simulink library "Mech_Hydro_Elec_Multibody_Lib"  (R2021b)
settings: Solver=ode45  StartTime=0.0  StopTime=10.0  RelTol=1e-3  EnableMultiTasking=on
libraries: fl_ps_legacy_lib x27, fl_lib x24, mech_hydro_forcesPS_lib x21, sm_lib x15, $bdroot x4
(part 2 of 2)

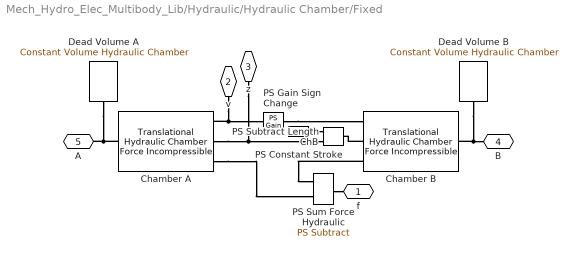
== system Mech_Hydro_Elec_Multibody_Lib/Hydraulic/Hydraulic Chamber/Fixed ==
  Chamber A : mech_hydro_forcesPS_lib/Hydraulic/Translational Hydraulic Chamber Force Incompressible  area=area_A m^2  q_specify=off  q_priority=None  q=0 m^3/s  q_nominal_specify=off  q_nominal_unit=m^3/s  q_nominal_value=1
      settings: InternalSimscapePortConfiguration="{\"Bottom\":[],\"Left\":[{\"id\":\"velocity\",\"label\":\"v\",\"type\":\"input\"},{\"id\":\"position\",\"label\":\"p\",\"type\":\"input\"},{\"id\":\"force\",\"label\":\"f\",\"type\":\"output\"}],\"Right\":[{\"id\":\"A\",\"label\":\"A\",\"type\":\"foundation.hydraulic.hydraulic\"}],\"Top\":[]}"
  Chamber B : mech_hydro_forcesPS_lib/Hydraulic/Translational Hydraulic Chamber Force Incompressible  area=area_B m^2  q_specify=off  q_priority=None  q=0 m^3/s  q_nominal_specify=off  q_nominal_unit=m^3/s  q_nominal_value=1
      settings: InternalSimscapePortConfiguration="{\"Bottom\":[],\"Left\":[{\"id\":\"velocity\",\"label\":\"v\",\"type\":\"input\"},{\"id\":\"position\",\"label\":\"p\",\"type\":\"input\"},{\"id\":\"force\",\"label\":\"f\",\"type\":\"output\"}],\"Right\":[{\"id\":\"A\",\"label\":\"A\",\"type\":\"foundation.hydraulic.hydraulic\"}],\"Top\":[]}"
  Dead Volume A : fl_lib/Hydraulic/Hydraulic Elements/Constant Volume Hydraulic Chamber  ch_sp=1  wall_type=1  ch_volume=dead_vol_A m^3  d_in=1e-2 m  length=1 m  pr_r_coef=1.2e-12 m/Pa  time_const=0.01 s  k_sh=1.4  pressure_specify=off  pressure_priority=High  pressure=0 Pa  pressure_nominal_specify=off  pressure_nominal_unit=Pa  pressure_nominal_value=1  diameter_incr_specify=off  diameter_incr_priority=High  diameter_incr=0 m  diameter_incr_nominal_specify=off  diameter_incr_nominal_unit=m  diameter_incr_nominal_value=1  flow_rate_specify=off  flow_rate_priority=None  flow_rate=0.001 m^3/s  flow_rate_nominal_specify=off  flow_rate_nominal_unit=m^3/s  flow_rate_nominal_value=1
      settings: SourceProductBaseCode=SS  InternalSimscapePortConfiguration="{\"Bottom\":[],\"Left\":[{\"id\":\"A\",\"label\":\"\",\"type\":\"foundation.hydraulic.hydraulic\"}],\"Right\":[],\"Top\":[]}"
  Dead Volume B : fl_lib/Hydraulic/Hydraulic Elements/Constant Volume Hydraulic Chamber  ch_sp=1  wall_type=1  ch_volume=dead_vol_B m^3  d_in=1e-2 m  length=1 m  pr_r_coef=1.2e-12 m/Pa  time_const=0.01 s  k_sh=1.4  pressure_specify=off  pressure_priority=High  pressure=0 Pa  pressure_nominal_specify=off  pressure_nominal_unit=Pa  pressure_nominal_value=1  diameter_incr_specify=off  diameter_incr_priority=High  diameter_incr=0 m  diameter_incr_nominal_specify=off  diameter_incr_nominal_unit=m  diameter_incr_nominal_value=1  flow_rate_specify=off  flow_rate_priority=None  flow_rate=0.001 m^3/s  flow_rate_nominal_specify=off  flow_rate_nominal_unit=m^3/s  flow_rate_nominal_value=1
      settings: SourceProductBaseCode=SS  InternalSimscapePortConfiguration="{\"Bottom\":[],\"Left\":[{\"id\":\"A\",\"label\":\"\",\"type\":\"foundation.hydraulic.hydraulic\"}],\"Right\":[],\"Top\":[]}"
  PS Constant Stroke : fl_lib/Physical Signals/Sources/PS Constant  constant=hs_stroke
  PS Gain Sign Change : fl_ps_legacy_lib/Legacy Physical Signals/Functions/PS Gain  gain=-1
  PS Subtract Length ChB : fl_ps_legacy_lib/Legacy Physical Signals/Functions/PS Subtract
      settings: SourceProductBaseCode=SS
  PS Sum Force Hydraulic : fl_ps_legacy_lib/Legacy Physical Signals/Functions/PS Subtract
      settings: SourceProductBaseCode=SS
  f : PMIOPort  Side=Right
  v : PMIOPort  Port=2  Side=Left
  z : PMIOPort  Port=3  Side=Left
  B : PMIOPort  Port=4  Side=Right
  A : PMIOPort  Port=5  Side=Left
  connections:
  PS Sum Force Hydraulic/RConn1 -- f/RConn1
  Chamber B/LConn2 -- PS Subtract Length ChB/RConn1
  Dead Volume B/LConn1 -- B/RConn1 -- Chamber B/RConn1
  PS Constant Stroke/RConn1 -- PS Subtract Length ChB/LConn1
  Chamber B/LConn3 -- PS Sum Force Hydraulic/LConn1
  PS Gain Sign Change/RConn1 -- Chamber B/LConn1
  Chamber A/LConn3 -- PS Sum Force Hydraulic/LConn2
  Dead Volume A/LConn1 -- A/RConn1 -- Chamber A/RConn1
  v/RConn1 -- PS Gain Sign Change/LConn1 -- Chamber A/LConn1
  z/RConn1 -- PS Subtract Length ChB/LConn2 -- Chamber A/LConn2

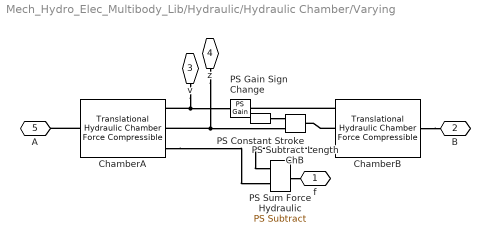
== system Mech_Hydro_Elec_Multibody_Lib/Hydraulic/Hydraulic Chamber/Varying ==
  ChamberA : mech_hydro_forcesPS_lib/Hydraulic/Translational Hydraulic Chamber Force Compressible  area=area_A m^2  V_dead=dead_vol_A m^3  k_sh=1.4  initial_pressure=0 Pa
      settings: InternalSimscapePortConfiguration="{\"Bottom\":[],\"Left\":[{\"id\":\"velocity\",\"label\":\"v\",\"type\":\"input\"},{\"id\":\"position\",\"label\":\"p\",\"type\":\"input\"},{\"id\":\"force\",\"label\":\"f\",\"type\":\"output\"}],\"Right\":[{\"id\":\"A\",\"label\":\"A\",\"type\":\"foundation.hydraulic.hydraulic\"}],\"Top\":[]}"
  ChamberB : mech_hydro_forcesPS_lib/Hydraulic/Translational Hydraulic Chamber Force Compressible  area=area_B m^2  V_dead=dead_vol_B m^3  k_sh=1.4  initial_pressure=0 Pa
      settings: InternalSimscapePortConfiguration="{\"Bottom\":[],\"Left\":[{\"id\":\"velocity\",\"label\":\"v\",\"type\":\"input\"},{\"id\":\"position\",\"label\":\"p\",\"type\":\"input\"},{\"id\":\"force\",\"label\":\"f\",\"type\":\"output\"}],\"Right\":[{\"id\":\"A\",\"label\":\"A\",\"type\":\"foundation.hydraulic.hydraulic\"}],\"Top\":[]}"
  PS Constant Stroke : fl_lib/Physical Signals/Sources/PS Constant  constant=hs_stroke
  PS Gain Sign Change : fl_ps_legacy_lib/Legacy Physical Signals/Functions/PS Gain  gain=-1
  PS Subtract Length ChB : fl_ps_legacy_lib/Legacy Physical Signals/Functions/PS Subtract
      settings: SourceProductBaseCode=SS
  PS Sum Force Hydraulic : fl_ps_legacy_lib/Legacy Physical Signals/Functions/PS Subtract
      settings: SourceProductBaseCode=SS
  f : PMIOPort  Side=Right
  B : PMIOPort  Port=2  Side=Right
  v : PMIOPort  Port=3  Side=Left
  z : PMIOPort  Port=4  Side=Left
  A : PMIOPort  Port=5  Side=Left
  connections:
  ChamberA/RConn1 -- A/RConn1
  ChamberA/LConn3 -- PS Sum Force Hydraulic/LConn2
  ChamberB/LConn3 -- PS Sum Force Hydraulic/LConn1
  ChamberB/RConn1 -- B/RConn1
  PS Sum Force Hydraulic/RConn1 -- f/RConn1
  v/RConn1 -- ChamberA/LConn1 -- PS Gain Sign Change/LConn1
  z/RConn1 -- ChamberA/LConn2 -- PS Subtract Length ChB/LConn2
  PS Constant Stroke/RConn1 -- PS Subtract Length ChB/LConn1
  ChamberB/LConn1 -- PS Gain Sign Change/RConn1
  ChamberB/LConn2 -- PS Subtract Length ChB/RConn1

== system Mech_Hydro_Elec_Multibody_Lib/Hydraulic/Hydraulic Chamber SA/Fixed ==
  Chamber A : mech_hydro_forcesPS_lib/Hydraulic/Translational Hydraulic Chamber Force Incompressible  area=area_A m^2  q_specify=off  q_priority=None  q=0 m^3/s  q_nominal_specify=off  q_nominal_unit=m^3/s  q_nominal_value=1
      settings: InternalSimscapePortConfiguration="{\"Bottom\":[],\"Left\":[{\"id\":\"velocity\",\"label\":\"v\",\"type\":\"input\"},{\"id\":\"position\",\"label\":\"p\",\"type\":\"input\"},{\"id\":\"force\",\"label\":\"f\",\"type\":\"output\"}],\"Right\":[{\"id\":\"A\",\"label\":\"A\",\"type\":\"foundation.hydraulic.hydraulic\"}],\"Top\":[]}"
  Dead Volume A : fl_lib/Hydraulic/Hydraulic Elements/Constant Volume Hydraulic Chamber  ch_sp=1  wall_type=1  ch_volume=dead_vol_A m^3  d_in=1e-2 m  length=1 m  pr_r_coef=1.2e-12 m/Pa  time_const=0.01 s  k_sh=1.4  pressure_specify=off  pressure_priority=High  pressure=0 Pa  pressure_nominal_specify=off  pressure_nominal_unit=Pa  pressure_nominal_value=1  diameter_incr_specify=off  diameter_incr_priority=High  diameter_incr=0 m  diameter_incr_nominal_specify=off  diameter_incr_nominal_unit=m  diameter_incr_nominal_value=1  flow_rate_specify=off  flow_rate_priority=None  flow_rate=0.001 m^3/s  flow_rate_nominal_specify=off  flow_rate_nominal_unit=m^3/s  flow_rate_nominal_value=1
      settings: SourceProductBaseCode=SS  InternalSimscapePortConfiguration="{\"Bottom\":[],\"Left\":[{\"id\":\"A\",\"label\":\"\",\"type\":\"foundation.hydraulic.hydraulic\"}],\"Right\":[],\"Top\":[]}"
  PS Gain : fl_ps_legacy_lib/Legacy Physical Signals/Functions/PS Gain  gain=-1
  f : PMIOPort  Side=Right
  v : PMIOPort  Port=2  Side=Left
  z : PMIOPort  Port=3  Side=Left
  A : PMIOPort  Port=4  Side=Left
  connections:
  z/RConn1 -- Chamber A/LConn2
  v/RConn1 -- Chamber A/LConn1
  Chamber A/RConn1 -- A/RConn1 -- Dead Volume A/LConn1
  Chamber A/LConn3 -- PS Gain/LConn1
  PS Gain/RConn1 -- f/RConn1

== system Mech_Hydro_Elec_Multibody_Lib/Hydraulic/Hydraulic Chamber SA/Varying ==
  ChamberA : mech_hydro_forcesPS_lib/Hydraulic/Translational Hydraulic Chamber Force Compressible  area=area_A m^2  V_dead=dead_vol_A m^3  k_sh=1.4  initial_pressure=0 Pa
      settings: InternalSimscapePortConfiguration="{\"Bottom\":[],\"Left\":[{\"id\":\"velocity\",\"label\":\"v\",\"type\":\"input\"},{\"id\":\"position\",\"label\":\"p\",\"type\":\"input\"},{\"id\":\"force\",\"label\":\"f\",\"type\":\"output\"}],\"Right\":[{\"id\":\"A\",\"label\":\"A\",\"type\":\"foundation.hydraulic.hydraulic\"}],\"Top\":[]}"
  PS Gain : fl_ps_legacy_lib/Legacy Physical Signals/Functions/PS Gain  gain=-1
  f : PMIOPort  Side=Right
  v : PMIOPort  Port=2  Side=Left
  z : PMIOPort  Port=3  Side=Left
  A : PMIOPort  Port=4  Side=Left
  connections:
  z/RConn1 -- ChamberA/LConn2
  v/RConn1 -- ChamberA/LConn1
  PS Gain/RConn1 -- f/RConn1
  ChamberA/LConn3 -- PS Gain/LConn1
  ChamberA/RConn1 -- A/RConn1

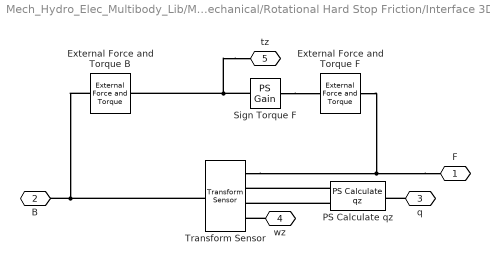
== system Mech_Hydro_Elec_Multibody_Lib/Mechanical/Rotational Hard Stop Friction/Interface 3D-1D ==
  External Force and Torque B : sm_lib/Forces and Torques/External Force and Torque  ForceResolutionFrame=AttachedFrame  EnableForceX=off  EnableForceY=off  EnableForceZ=off  EnableForce=off  TorqueResolutionFrame=AttachedFrame  EnableTorqueX=off  EnableTorqueY=off  EnableTorqueZ=on  EnableTorque=off
  External Force and Torque F : sm_lib/Forces and Torques/External Force and Torque  ForceResolutionFrame=AttachedFrame  EnableForceX=off  EnableForceY=off  EnableForceZ=off  EnableForce=off  TorqueResolutionFrame=AttachedFrame  EnableTorqueX=off  EnableTorqueY=off  EnableTorqueZ=on  EnableTorque=off
  PS Calculate qz : mech_hydro_forcesPS_lib/Math/PS Calculate qz
      settings: InternalSimscapePortConfiguration="{\"Bottom\":[],\"Left\":[{\"id\":\"q\",\"label\":\"q\",\"type\":\"input\"},{\"id\":\"axs\",\"label\":\"axs\",\"type\":\"input\"}],\"Right\":[{\"id\":\"qz\",\"label\":\"qz\",\"type\":\"output\"}],\"Top\":[]}"
  Sign Torque F : fl_ps_legacy_lib/Legacy Physical Signals/Functions/PS Gain  gain=-1
  Transform Sensor : sm_lib/Frames and Transforms/Transform Sensor  MeasurementFrame=Base  SenseAngle=on  SenseAxis=on  SenseAngle1=off  SenseAngle2=off  SenseAngle3=off  SenseQ=off  SenseR=off  SenseOmegaX=off  SenseOmegaY=off  SenseOmegaZ=on  SenseOmega1=off  SenseOmega2=off  SenseOmega3=off  SenseQDot=off  SenseRDot=off  SenseAlphaX=off  SenseAlphaY=off  SenseAlphaZ=off  SenseAlpha1=off  SenseAlpha2=off  SenseAlpha3=off  SenseQDDot=off  SenseRDDot=off  SenseX=off  SenseY=off  SenseZ=off  SenseRad=off  SenseAzim=off  SenseDist=off  SenseInc=off  SenseXDot=off  SenseYDot=off  SenseZDot=off  SenseRadDot=off  SenseAzimDot=off  SenseDistDot=off  SenseIncDot=off  SenseXDDot=off  SenseYDDot=off  SenseZDDot=off  SenseRadDDot=off  SenseAzimDDot=off  SenseDistDDot=off  SenseIncDDot=off
  F : PMIOPort  Side=Right
  B : PMIOPort  Port=2  Side=Left
  q : PMIOPort  Port=3  Side=Left
  wz : PMIOPort  Port=4  Side=Left
  tz : PMIOPort  Port=5  Side=Right
  connections:
  q/RConn1 -- PS Calculate qz/RConn1
  PS Calculate qz/LConn2 -- Transform Sensor/RConn3
  PS Calculate qz/LConn1 -- Transform Sensor/RConn2
  tz/RConn1 -- External Force and Torque B/LConn1 -- Sign Torque F/LConn1
  Sign Torque F/RConn1 -- External Force and Torque F/LConn1
  wz/RConn1 -- Transform Sensor/RConn4
  External Force and Torque B/RConn1 -- B/RConn1 -- Transform Sensor/LConn1
  F/RConn1 -- Transform Sensor/RConn1 -- External Force and Torque F/RConn1

== system Mech_Hydro_Elec_Multibody_Lib/Mechanical/Translational Hard Stop Friction/Interface 3D-1D ==
  External Force and Torque B : sm_lib/Forces and Torques/External Force and Torque  ForceResolutionFrame=AttachedFrame  EnableForceX=off  EnableForceY=off  EnableForceZ=on  EnableForce=off  TorqueResolutionFrame=AttachedFrame  EnableTorqueX=off  EnableTorqueY=off  EnableTorqueZ=off  EnableTorque=off
  External Force and Torque F : sm_lib/Forces and Torques/External Force and Torque  ForceResolutionFrame=AttachedFrame  EnableForceX=off  EnableForceY=off  EnableForceZ=on  EnableForce=off  TorqueResolutionFrame=AttachedFrame  EnableTorqueX=off  EnableTorqueY=off  EnableTorqueZ=off  EnableTorque=off
  Sign Force F : fl_ps_legacy_lib/Legacy Physical Signals/Functions/PS Gain  gain=-1
  Transform Sensor : sm_lib/Frames and Transforms/Transform Sensor  MeasurementFrame=Base  SenseAngle=off  SenseAxis=off  SenseAngle1=off  SenseAngle2=off  SenseAngle3=off  SenseQ=off  SenseR=off  SenseOmegaX=off  SenseOmegaY=off  SenseOmegaZ=off  SenseOmega1=off  SenseOmega2=off  SenseOmega3=off  SenseQDot=off  SenseRDot=off  SenseAlphaX=off  SenseAlphaY=off  SenseAlphaZ=off  SenseAlpha1=off  SenseAlpha2=off  SenseAlpha3=off  SenseQDDot=off  SenseRDDot=off  SenseX=off  SenseY=off  SenseZ=on  SenseRad=off  SenseAzim=off  SenseDist=off  SenseInc=off  SenseXDot=off  SenseYDot=off  SenseZDot=on  SenseRadDot=off  SenseAzimDot=off  SenseDistDot=off  SenseIncDot=off  SenseXDDot=off  SenseYDDot=off  SenseZDDot=off  SenseRadDDot=off  SenseAzimDDot=off  SenseDistDDot=off  SenseIncDDot=off
  F : PMIOPort  Side=Right
  B : PMIOPort  Port=2  Side=Left
  z : PMIOPort  Port=3  Side=Left
  vz : PMIOPort  Port=4  Side=Left
  fz : PMIOPort  Port=5  Side=Right
  connections:
  Transform Sensor/RConn1 -- F/RConn1 -- External Force and Torque F/RConn1
  Transform Sensor/LConn1 -- B/RConn1 -- External Force and Torque B/RConn1
  z/RConn1 -- Transform Sensor/RConn2
  vz/RConn1 -- Transform Sensor/RConn3
  Sign Force F/RConn1 -- External Force and Torque F/LConn1
  Sign Force F/LConn1 -- External Force and Torque B/LConn1 -- fz/RConn1
